simulink subsystem "rss_SplyVltgLoLvl1Dia"  (R2023a)
settings: Solver=VariableStepAuto  StartTime=0.0  StopTime=10.0  RelTol=1e-3
undefined symbols (not defined in the file): Cdbl_uSplyVltgMaxVal, ENM_TYPE_FALT, Gu16_ctSplyVltgLoLvl1ConfCnt_C, Gu16_ctSplyVltgLoLvl1RcvyCnt_C, Gu16_uSplyVltgLoLvl1ConfTrs_C, Gu16_uSplyVltgLoLvl1RcvyTrs_C
libraries: vhit_control_library x1, lib_fault_definiteness x1
settings Model: Creator=xiaoqiang.yuan  LastModifiedBy=xiaoqiang.yuan

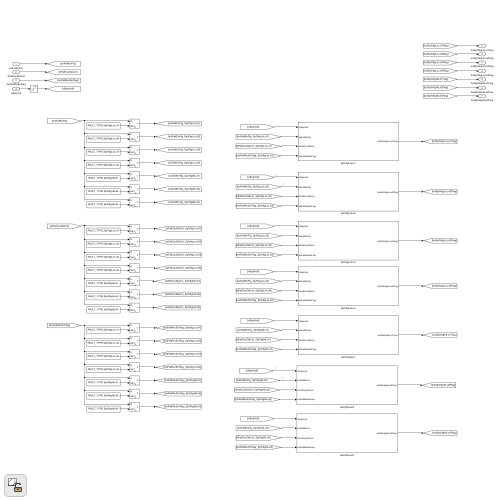
[thumbnail: Simulink's stored preview of the top-level diagram]
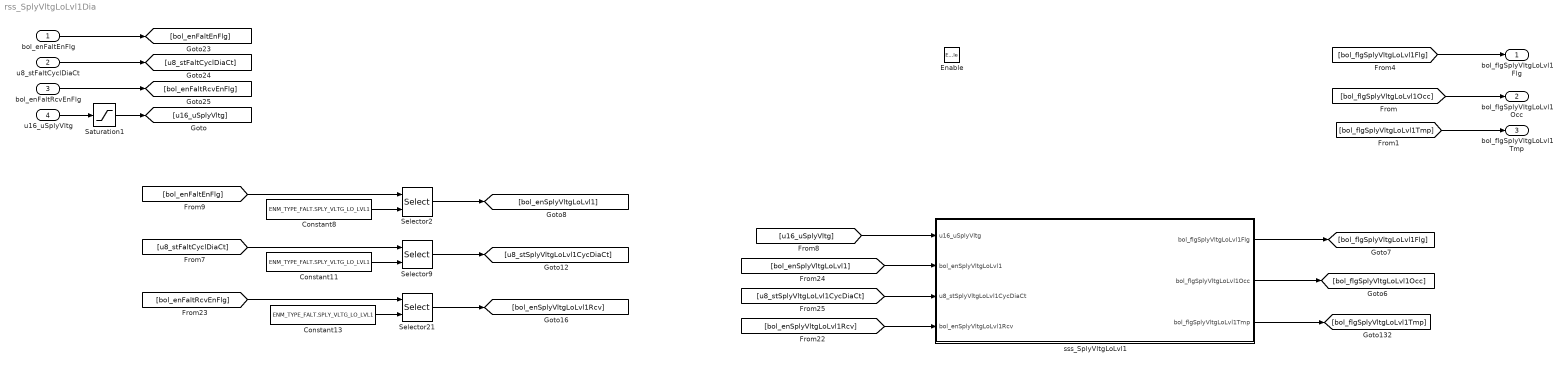
== system rss_SplyVltgLoLvl1Dia ==
  bol_enFaltEnFlg : Inport  OutDataTypeStr=boolean
  u8_stFaltCyclDiaCt : Inport  Port=2  OutDataTypeStr=uint8
  bol_enFaltRcvEnFlg : Inport  Port=3  OutDataTypeStr=boolean
  u16_uSplyVltg : Inport  Port=4  OutDataTypeStr=dt_Standardize_u16p15b0
  Enable : EnablePort
  Constant11 : Constant  Value=ENM_TYPE_FALT.SPLY_VLTG_LO_LVL1
  Constant13 : Constant  Value=ENM_TYPE_FALT.SPLY_VLTG_LO_LVL1
  Constant8 : Constant  Value=ENM_TYPE_FALT.SPLY_VLTG_LO_LVL1
  Saturation1 : Saturate  UpperLimit=Cdbl_uSplyVltgMaxVal  LowerLimit=0
  Selector2 : Selector  IndexMode=Zero-based  InputPortWidth=Cdbl_numFaltDiaNum  IndexOptions=Index vector (port)  Indices=[1 3]  OutputSizes=1
  Selector21 : Selector  IndexMode=Zero-based  InputPortWidth=Cdbl_numFaltDiaNum  IndexOptions=Index vector (port)  Indices=[1 3]  OutputSizes=1
  Selector9 : Selector  IndexMode=Zero-based  InputPortWidth=Cdbl_numFaltDiaNum  IndexOptions=Index vector (port)  Indices=[1 3]  OutputSizes=1
  sss_SplyVltgLoLvl1 : Subsystem
  bol_flgSplyVltgLoLvl1Flg : Outport  OutDataTypeStr=boolean
  bol_flgSplyVltgLoLvl1Occ : Outport  Port=2  OutDataTypeStr=boolean
  bol_flgSplyVltgLoLvl1Tmp : Outport  Port=3  OutDataTypeStr=boolean
  wires:
  [bol_flgSplyVltgLoLvl1Flg] -> bol_flgSplyVltgLoLvl1Flg/1
  [u8_stSplyVltgLoLvl1CycDiaCt] -> sss_SplyVltgLoLvl1/3(u8_stSplyVltgLoLvl1CycDiaCt)
  [u16_uSplyVltg] -> sss_SplyVltgLoLvl1/1(u16_uSplyVltg)
  [bol_enSplyVltgLoLvl1Rcv] -> sss_SplyVltgLoLvl1/4(bol_enSplyVltgLoLvl1Rcv)
  Constant8/1 -> Selector2/2
  sss_SplyVltgLoLvl1/1(bol_flgSplyVltgLoLvl1Flg) -> [bol_flgSplyVltgLoLvl1Flg]
  [bol_enSplyVltgLoLvl1] -> sss_SplyVltgLoLvl1/2(bol_enSplyVltgLoLvl1)
  Selector2/1 -> [bol_enSplyVltgLoLvl1]
  [bol_enFaltEnFlg] -> Selector2/1
  bol_enFaltEnFlg/1 -> [bol_enFaltEnFlg]
  bol_enFaltRcvEnFlg/1 -> [bol_enFaltRcvEnFlg]
  u8_stFaltCyclDiaCt/1 -> [u8_stFaltCyclDiaCt]
  Selector9/1 -> [u8_stSplyVltgLoLvl1CycDiaCt]
  Constant11/1 -> Selector9/2
  [u8_stFaltCyclDiaCt] -> Selector9/1
  Constant13/1 -> Selector21/2
  Selector21/1 -> [bol_enSplyVltgLoLvl1Rcv]
  u16_uSplyVltg/1 -> Saturation1/1
  Saturation1/1 -> [u16_uSplyVltg]
  [bol_enFaltRcvEnFlg] -> Selector21/1
  sss_SplyVltgLoLvl1/2(bol_flgSplyVltgLoLvl1Occ) -> [bol_flgSplyVltgLoLvl1Occ]
  [bol_flgSplyVltgLoLvl1Occ] -> bol_flgSplyVltgLoLvl1Occ/1
  [bol_flgSplyVltgLoLvl1Tmp] -> bol_flgSplyVltgLoLvl1Tmp/1
  sss_SplyVltgLoLvl1/3(bol_flgSplyVltgLoLvl1Tmp) -> [bol_flgSplyVltgLoLvl1Tmp]

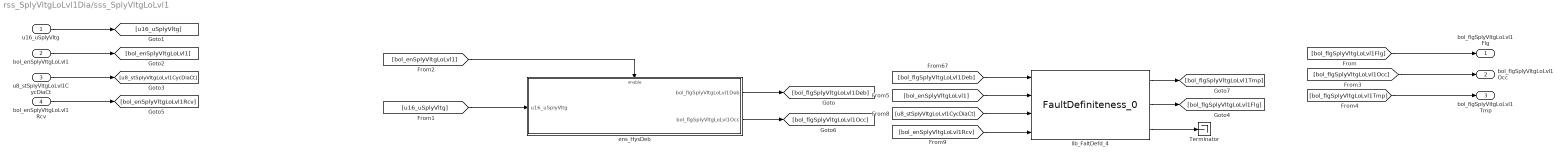
== system rss_SplyVltgLoLvl1Dia/sss_SplyVltgLoLvl1 ==
  u16_uSplyVltg : Inport
  bol_enSplyVltgLoLvl1 : Inport  Port=2
  u8_stSplyVltgLoLvl1CycDiaCt : Inport  Port=3
  bol_enSplyVltgLoLvl1Rcv : Inport  Port=4
  Terminator : Terminator
  ens_HysDeb : Subsystem
  lib_FaltDefd_4 : lib_fault_definiteness/FaultDefiniteness_0  lb_FaltWaitRecvCnt=Gu16_ctSplyVltgLoLvl1ConfCnt_C
  bol_flgSplyVltgLoLvl1Flg : Outport
  bol_flgSplyVltgLoLvl1Occ : Outport  Port=2
  bol_flgSplyVltgLoLvl1Tmp : Outport  Port=3
  wires:
  [bol_flgSplyVltgLoLvl1Tmp] -> bol_flgSplyVltgLoLvl1Tmp/1
  [bol_flgSplyVltgLoLvl1Occ] -> bol_flgSplyVltgLoLvl1Occ/1
  ens_HysDeb/2(bol_flgSplyVltgLoLvl1Occ) -> [bol_flgSplyVltgLoLvl1Occ]
  lib_FaltDefd_4/1 -> [bol_flgSplyVltgLoLvl1Tmp]
  lib_FaltDefd_4/2 -> [bol_flgSplyVltgLoLvl1Flg]
  lib_FaltDefd_4/3 -> Terminator/1
  [bol_enSplyVltgLoLvl1] -> ens_HysDeb/Enable
  [u16_uSplyVltg] -> ens_HysDeb/1(u16_uSplyVltg)
  ens_HysDeb/1(bol_flgSplyVltgLoLvl1Deb) -> [bol_flgSplyVltgLoLvl1Deb]
  bol_enSplyVltgLoLvl1Rcv/1 -> [bol_enSplyVltgLoLvl1Rcv]
  u8_stSplyVltgLoLvl1CycDiaCt/1 -> [u8_stSplyVltgLoLvl1CycDiaCt]
  bol_enSplyVltgLoLvl1/1 -> [bol_enSplyVltgLoLvl1]
  [bol_flgSplyVltgLoLvl1Flg] -> bol_flgSplyVltgLoLvl1Flg/1
  u16_uSplyVltg/1 -> [u16_uSplyVltg]
  [bol_enSplyVltgLoLvl1Rcv] -> lib_FaltDefd_4/4
  [u8_stSplyVltgLoLvl1CycDiaCt] -> lib_FaltDefd_4/3
  [bol_enSplyVltgLoLvl1] -> lib_FaltDefd_4/2
  [bol_flgSplyVltgLoLvl1Deb] -> lib_FaltDefd_4/1

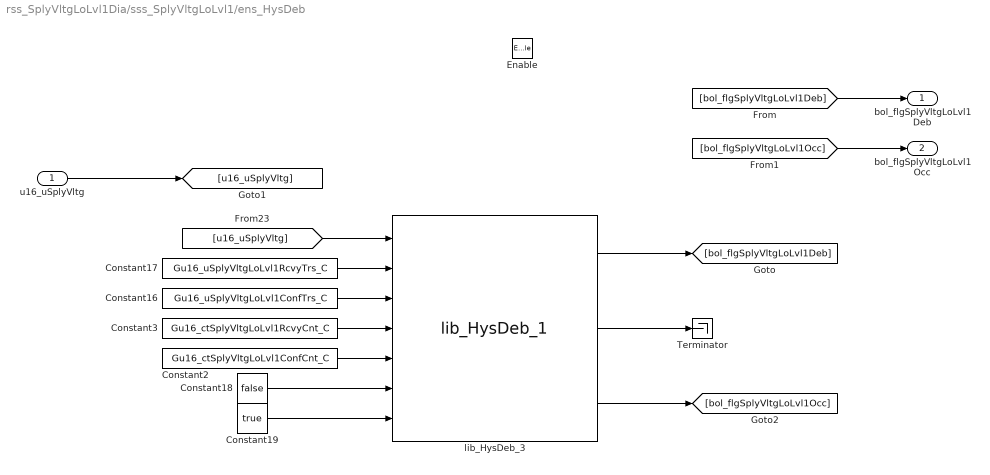
== system rss_SplyVltgLoLvl1Dia/sss_SplyVltgLoLvl1/ens_HysDeb ==
  u16_uSplyVltg : Inport
  Enable : EnablePort
  Constant16 : Constant  Value=Gu16_uSplyVltgLoLvl1ConfTrs_C
  Constant17 : Constant  Value=Gu16_uSplyVltgLoLvl1RcvyTrs_C
  Constant18 : Constant  Value=false  OutDataTypeStr=boolean
  Constant19 : Constant  Value=true  OutDataTypeStr=boolean
  Constant2 : Constant  Value=Gu16_ctSplyVltgLoLvl1ConfCnt_C
  Constant3 : Constant  Value=Gu16_ctSplyVltgLoLvl1RcvyCnt_C
  Terminator : Terminator
  lib_HysDeb_3 : vhit_control_library/lib_HysDeb_1  lb_parInitOutp=0
  bol_flgSplyVltgLoLvl1Deb : Outport
  bol_flgSplyVltgLoLvl1Occ : Outport  Port=2
  wires:
  [bol_flgSplyVltgLoLvl1Occ] -> bol_flgSplyVltgLoLvl1Occ/1
  lib_HysDeb_3/3 -> [bol_flgSplyVltgLoLvl1Occ]
  lib_HysDeb_3/2 -> Terminator/1
  Constant17/1 -> lib_HysDeb_3/2
  Constant16/1 -> lib_HysDeb_3/3
  Constant3/1 -> lib_HysDeb_3/4
  Constant2/1 -> lib_HysDeb_3/5
  lib_HysDeb_3/1 -> [bol_flgSplyVltgLoLvl1Deb]
  Constant19/1 -> lib_HysDeb_3/7
  Constant18/1 -> lib_HysDeb_3/6
  [u16_uSplyVltg] -> lib_HysDeb_3/1
  u16_uSplyVltg/1 -> [u16_uSplyVltg]
  [bol_flgSplyVltgLoLvl1Deb] -> bol_flgSplyVltgLoLvl1Deb/1
